simulink model "quadrotor_DRF"  (Simulink 9.1)
settings: Solver=ode4  StartTime=0.0  StopTime=inf  FixedStep=dt_simu  RelTol=1e-3
InitFcn:
  | init
model workspace: external: MAT-File model_workspace.mat (data not in the file)
values from neighbouring files (symbols this model uses):
  X0 = [phi0 theta0 0 p0 q0 r0]'    [init.m]
settings Model: Creator=Sihao  LastModifiedBy=samsun  EnablePacing=on
settings DataIOCC: LimitDataPoints=on
settings DebuggingCC: UnderspecifiedInitializationDetection=Simplified  MergeDetectMultiDrivingBlocksExec=error  SolverPrmCheckMsg=warning  AllowSymbolicDim=off
settings GRTTargetCC: GeneratePreprocessorConditionals=Disable all  CombineOutputUpdateFcns=on  GRTInterface=off
settings ConfigComp: CovSFcnEnable=off
settings SimscapeCC: SimscapeNormalizeSystem=off
settings ConfigurationSet: Description=SimMechanics 2G

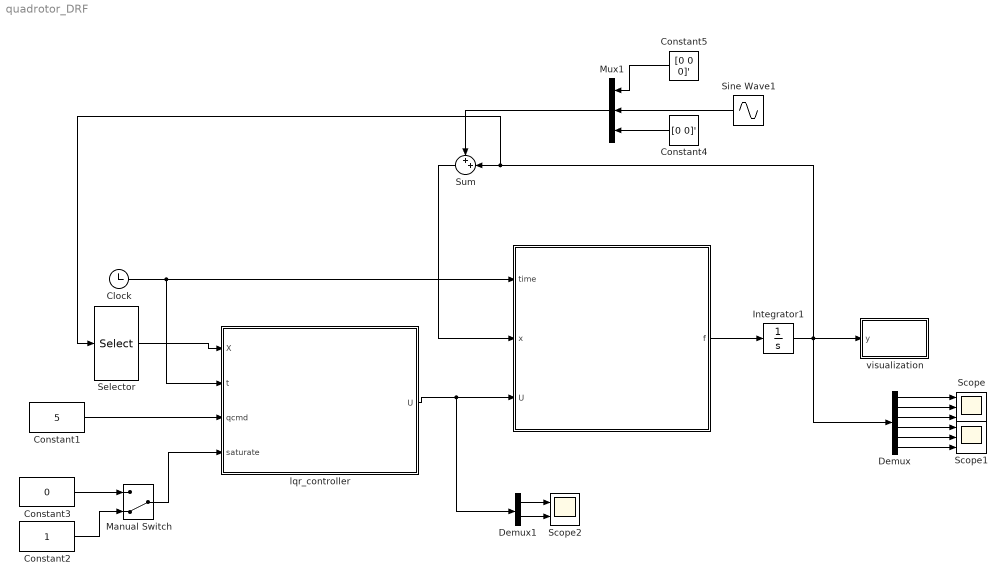
== system quadrotor_DRF ==
  " " : MATLAB Function  TreatAsAtomicUnit=on
  Clock : Clock
  Constant1 : Constant  Value=5
  Constant2 : Constant
  Constant3 : Constant  Value=0
  Constant4 : Constant  Value=[0 0]'
  Constant5 : Constant  Value=[0 0 0]'
  Demux : Demux  Outputs=6
  Demux1 : Demux  Outputs=2
  Integrator1 : Integrator  InitialCondition=X0
  Manual Switch : ManualSwitch  CurrentSetting=0
  Mux1 : Mux  Inputs=3
  Scope : Scope  NumInputPorts=3
  Scope1 : Scope  NumInputPorts=3
  Scope2 : Scope  NumInputPorts=2
  Selector : Selector  InputPortWidth=6  IndexOptions=Index vector (dialog)  Indices=[4 5 6]  OutputSizes=1
  Sine Wave1 : Sin  Amplitude=0.00  SampleTime=0
  Sum : Sum  Inputs=++|
  lqr_controller : MATLAB Function  TreatAsAtomicUnit=on
  visualization : Subsystem
  wires:
  " "/1(f) -> Integrator1/1
  Clock/1 -> lqr_controller/2(t), " "/1(time)
  lqr_controller/1(U) -> Demux1/1, " "/3(U)
  Constant1/1 -> lqr_controller/3(qcmd)
  Demux/1 -> Scope/1
  Demux/2 -> Scope/2
  Demux/3 -> Scope/3
  Constant3/1 -> Manual Switch/1
  Constant2/1 -> Manual Switch/2
  Manual Switch/1 -> lqr_controller/4(saturate)
  Demux1/2 -> Scope2/2
  Demux1/1 -> Scope2/1
  Sum/1 -> " "/2(x)
  Integrator1/1 -> Selector/1, Sum/2, visualization/1(y), Demux/1
  Sine Wave1/1 -> Mux1/2
  Constant5/1 -> Mux1/1
  Selector/1 -> lqr_controller/1(X)
  Constant4/1 -> Mux1/3
  Demux/4 -> Scope1/1
  Demux/5 -> Scope1/2
  Demux/6 -> Scope1/3
  Mux1/1 -> Sum/1

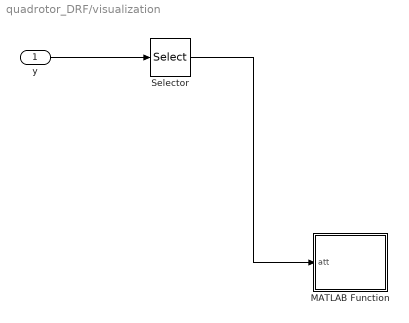
== system quadrotor_DRF/visualization ==
  y : Inport
  MATLAB Function : MATLAB Function  TreatAsAtomicUnit=on
  Selector : Selector  InputPortWidth=6  IndexOptions=Index vector (dialog)  Indices=[1 2 3]  OutputSizes=1
  wires:
  y/1 -> Selector/1
  Selector/1 -> MATLAB Function/1(att)

== matlab function   ==
  data: f output double; time input double; x input double; U input double; param parameter Bus: param_bus
function f = model_2D_quad(time,x,U,param)
%State space model of quadrotor

if time > 1.2  
    time = time;
end
%% Variable allocation
phi = x(1);
theta = x(2);
psi = x(3);
p = x(4);
q = x(5);
r = x(6);

u1 = U(1);
u2 = U(2);

Ix = param.Ix; Iy = param.Iy; Iz = param.Iz; Ip = param.Ip;
k = param.k; t = param.t; b = param.b; l = param.l; gamma = param.gamma;

f = zeros(6,1);

f(1) = p + tan(theta)*(q*sin(phi)+r*cos(phi));
f(2) = q*cos(phi)-r*sin(phi);
f(3) = (q*sin(phi)+r*cos(phi))/cos(theta);
f(4) = ((Iy-Iz)*q*r - Ip*q*(u1+u2) + k*b*(u1^2-u2^2))/Ix;
f(5) = ((Iz-Ix)*p*r + Ip*p*(u1+u2) + k*l*(u1^2-u2^2))/Iy;
f(6) = (-gamma*r + t*(u1^2+u2^2) + (Ix-Iy)*p*q)/Iz;

end

== matlab function lqr_controller ==
  data: X input double; U output double; t input double; qcmd input double; lqr_data parameter Bus: lqr_data_bus; saturate input double
function U = control_DRF_lqr(X,t,qcmd,lqr_data,saturate)

U = zeros(2,1);
% 
[~,j] = min(abs(lqr_data.X(2,:)-qcmd));

k = j;

K = lqr_data.K(:,:,k);
p0 = lqr_data.X(1,k);
q0 = lqr_data.X(2,k);
r0 = lqr_data.X(3,k);

X_ref = [p0 q0 r0]';
Ufb = K*(X_ref - X);
% Ufb = zeros(2,1);

u1 = lqr_data.X(4,k) + Ufb(1);
u2 = lqr_data.X(5,k) + Ufb(2);

u1max = inf;
u2max = inf;
if saturate == 1
    u1max = lqr_data.X(4,j); 
%     u1 = u1max;  % front rotor jammed!!
%     u2max = lqr_data.X(5,j);
end

U(1) = min(u1max,u1);
U(2) = min(u2max,u2);
end

== matlab function visualization/MATLAB Function ==
  settings: updateMethod=DISCRETE  sampleTime=3*dt_simu
  data: att input double
function fcn(att)

phi = att(1);
theta = att(2);
yaw = att(3);

t = get(gca,'Children');
t = t(1);

S = makehgtform('translate',[0 0 0]);
Rz = makehgtform('zrotate',yaw);
Ry = makehgtform('yrotate',theta);
Rx = makehgtform('xrotate',phi);

set(t,'Matrix',S*Rz*Ry*Rx);
% set(t,'Matrix',S);
drawnow

end
